simulink model "final_model"  (Simulink 10.0)
settings: Solver=VariableStepAuto  StartTime=0.0  StopTime=0.1  RelTol=1e-3
values from neighbouring files (symbols this model uses):
  Cth1 = 2.995e-4    (= 0.0002995)    [Initialization_naireeta.m]
  Cth2 = 0.0044    [Initialization_naireeta.m]
  Cth3 = 0.00376    [Initialization_naireeta.m]
  Irate = 10    [Initialization_naireeta.m]
  J = 1440    [Initialization_naireeta.m]
  Llrp = 0.00824    [Initialization_naireeta.m]
  Lls = 0.00103    [Initialization_naireeta.m]
  LM = 0.00639    [Initialization_naireeta.m]
  P = 4    [Initialization_naireeta.m]
  rrp = 2.25    [Initialization_naireeta.m]
  rs = 0.4    [Initialization_naireeta.m]
  Rth1 = 0.0850    (= 0.085)    [Initialization_naireeta.m]
  Rth2 = 0.353    [Initialization_naireeta.m]
  Rth3 = 0.7321    [Initialization_naireeta.m]
  Ts = 1e-6    (= 1e-06)    [Initialization_naireeta.m]
libraries: powerlib x135, powerlib_meascontrol x3, simulink x1
(part 2 of 2)

== system final_model/Thermal /Subsystem8 ==
  Ploss : Inport
  Ta : Inport  Port=2
  Controlled Current Source : powerlib/Electrical Sources/Controlled Current Source  Initialize=on  Source_Type=AC  Amplitude=0  Phase=0  Frequency=0  Measurements=None
      settings: SourceProductName=Simscape Electrical
  Controlled Voltage Source : powerlib/Electrical Sources/Controlled Voltage Source  Initialize=on  Source_Type=AC  Amplitude=0  Phase=0  Frequency=0  Measurements=None
      settings: SourceProductName=Simscape Electrical
  Series RLC Branch : powerlib/Elements/Series RLC Branch  LConnTagsString=__new0  RConnTagsString=__new0  BranchType=R  Resistance=Rth1  Inductance=1e-3  SetiL0=off  InitialCurrent=0  Capacitance=1e-6  Setx0=off  InitialVoltage=0  Measurements=None
      settings: SourceProductName=Simscape Electrical
  Series RLC Branch1 : powerlib/Elements/Series RLC Branch  LConnTagsString=__new0  RConnTagsString=__new0  BranchType=C  Resistance=1  Inductance=1e-3  SetiL0=off  InitialCurrent=0  Capacitance=Cth1  Setx0=off  InitialVoltage=0  Measurements=None
      settings: SourceProductName=Simscape Electrical
  Series RLC Branch2 : powerlib/Elements/Series RLC Branch  LConnTagsString=__new0  RConnTagsString=__new0  BranchType=R  Resistance=Rth2  Inductance=1e-3  SetiL0=off  InitialCurrent=0  Capacitance=1e-6  Setx0=off  InitialVoltage=0  Measurements=None
      settings: SourceProductName=Simscape Electrical
  Series RLC Branch3 : powerlib/Elements/Series RLC Branch  LConnTagsString=__new0  RConnTagsString=__new0  BranchType=C  Resistance=1  Inductance=1e-3  SetiL0=off  InitialCurrent=0  Capacitance=Cth2  Setx0=off  InitialVoltage=0  Measurements=None
      settings: SourceProductName=Simscape Electrical
  Series RLC Branch4 : powerlib/Elements/Series RLC Branch  LConnTagsString=__new0  RConnTagsString=__new0  BranchType=R  Resistance=Rth3  Inductance=1e-3  SetiL0=off  InitialCurrent=0  Capacitance=1e-6  Setx0=off  InitialVoltage=0  Measurements=None
      settings: SourceProductName=Simscape Electrical
  Series RLC Branch5 : powerlib/Elements/Series RLC Branch  LConnTagsString=__new0  RConnTagsString=__new0  BranchType=C  Resistance=1  Inductance=1e-3  SetiL0=off  InitialCurrent=0  Capacitance=Cth3  Setx0=off  InitialVoltage=0  Measurements=None
      settings: SourceProductName=Simscape Electrical
  Voltage Measurement : powerlib/Measurements/Voltage Measurement  PhasorSimulation=off  OutputType=Complex  PSBequivalent=0
      settings: SourceProductName=Simscape Electrical
  "TJ1 " : Outport
  wires:
  Ploss/1 -> Controlled Current Source/1
  Ta/1 -> Controlled Voltage Source/1
  Voltage Measurement/1 -> "TJ1 "/1
  connections:
  Series RLC Branch/LConn1 -- Series RLC Branch1/LConn1 -- Controlled Current Source/RConn1
  Series RLC Branch/RConn1 -- Voltage Measurement/LConn1 -- Series RLC Branch2/LConn1 -- Series RLC Branch3/LConn1 -- Series RLC Branch1/RConn1
  Controlled Voltage Source/LConn1 -- Voltage Measurement/LConn2 -- Controlled Current Source/LConn1
  Series RLC Branch4/LConn1 -- Series RLC Branch5/LConn1 -- Series RLC Branch2/RConn1 -- Series RLC Branch3/RConn1
  Series RLC Branch4/RConn1 -- Controlled Voltage Source/RConn1 -- Series RLC Branch5/RConn1

== system final_model/Thermal /Subsystem9 ==
  Ploss : Inport
  Ta : Inport  Port=2
  Controlled Current Source : powerlib/Electrical Sources/Controlled Current Source  Initialize=on  Source_Type=AC  Amplitude=0  Phase=0  Frequency=0  Measurements=None
      settings: SourceProductName=Simscape Electrical
  Controlled Voltage Source : powerlib/Electrical Sources/Controlled Voltage Source  Initialize=on  Source_Type=AC  Amplitude=0  Phase=0  Frequency=0  Measurements=None
      settings: SourceProductName=Simscape Electrical
  Series RLC Branch : powerlib/Elements/Series RLC Branch  LConnTagsString=__new0  RConnTagsString=__new0  BranchType=R  Resistance=Rth1  Inductance=1e-3  SetiL0=off  InitialCurrent=0  Capacitance=1e-6  Setx0=off  InitialVoltage=0  Measurements=None
      settings: SourceProductName=Simscape Electrical
  Series RLC Branch1 : powerlib/Elements/Series RLC Branch  LConnTagsString=__new0  RConnTagsString=__new0  BranchType=C  Resistance=1  Inductance=1e-3  SetiL0=off  InitialCurrent=0  Capacitance=Cth1  Setx0=off  InitialVoltage=0  Measurements=None
      settings: SourceProductName=Simscape Electrical
  Series RLC Branch2 : powerlib/Elements/Series RLC Branch  LConnTagsString=__new0  RConnTagsString=__new0  BranchType=R  Resistance=Rth2  Inductance=1e-3  SetiL0=off  InitialCurrent=0  Capacitance=1e-6  Setx0=off  InitialVoltage=0  Measurements=None
      settings: SourceProductName=Simscape Electrical
  Series RLC Branch3 : powerlib/Elements/Series RLC Branch  LConnTagsString=__new0  RConnTagsString=__new0  BranchType=C  Resistance=1  Inductance=1e-3  SetiL0=off  InitialCurrent=0  Capacitance=Cth2  Setx0=off  InitialVoltage=0  Measurements=None
      settings: SourceProductName=Simscape Electrical
  Series RLC Branch4 : powerlib/Elements/Series RLC Branch  LConnTagsString=__new0  RConnTagsString=__new0  BranchType=R  Resistance=Rth3  Inductance=1e-3  SetiL0=off  InitialCurrent=0  Capacitance=1e-6  Setx0=off  InitialVoltage=0  Measurements=None
      settings: SourceProductName=Simscape Electrical
  Series RLC Branch5 : powerlib/Elements/Series RLC Branch  LConnTagsString=__new0  RConnTagsString=__new0  BranchType=C  Resistance=1  Inductance=1e-3  SetiL0=off  InitialCurrent=0  Capacitance=Cth3  Setx0=off  InitialVoltage=0  Measurements=None
      settings: SourceProductName=Simscape Electrical
  Voltage Measurement : powerlib/Measurements/Voltage Measurement  PhasorSimulation=off  OutputType=Complex  PSBequivalent=0
      settings: SourceProductName=Simscape Electrical
  "TJ1 " : Outport
  wires:
  Ploss/1 -> Controlled Current Source/1
  Ta/1 -> Controlled Voltage Source/1
  Voltage Measurement/1 -> "TJ1 "/1
  connections:
  Series RLC Branch/LConn1 -- Series RLC Branch1/LConn1 -- Controlled Current Source/RConn1
  Series RLC Branch/RConn1 -- Voltage Measurement/LConn1 -- Series RLC Branch2/LConn1 -- Series RLC Branch3/LConn1 -- Series RLC Branch1/RConn1
  Controlled Voltage Source/LConn1 -- Voltage Measurement/LConn2 -- Controlled Current Source/LConn1
  Series RLC Branch4/LConn1 -- Series RLC Branch5/LConn1 -- Series RLC Branch2/RConn1 -- Series RLC Branch3/RConn1
  Series RLC Branch4/RConn1 -- Controlled Voltage Source/RConn1 -- Series RLC Branch5/RConn1

== system final_model/IM /Dynamic model of IM/Electromagnetic Torque ==
  Add : Sum  Inputs=+-
  Gain : Gain  Gain=(3/2)*(P/2)
  Product : Product  RndMeth=Zero
  Product1 : Product  RndMeth=Zero
  tag scope: Te=global
  wires:
  Add/1 -> Gain/1
  [lamda_ds] -> Product/1
  [iqs] -> Product/2
  [lamda_qs] -> Product1/1
  [ids] -> Product1/2
  Product/1 -> Add/1
  Product1/1 -> Add/2
  Gain/1 -> [Te]

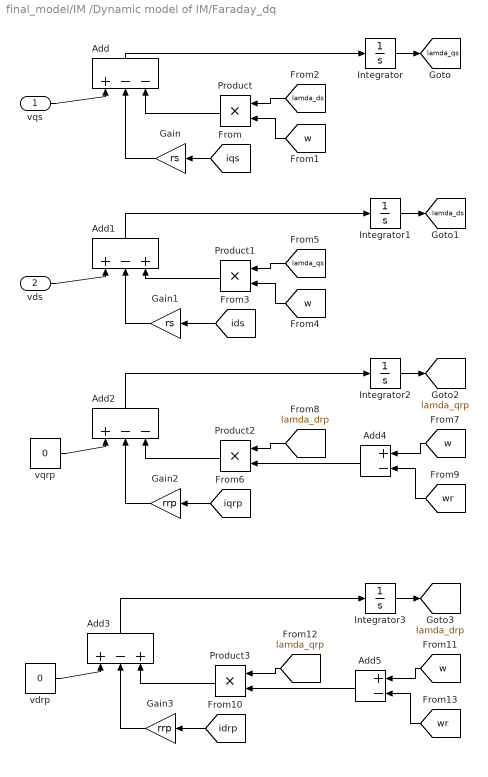
== system final_model/IM /Dynamic model of IM/Faraday_dq ==
  vqs : Inport
  vds : Inport  Port=2
  Add : Sum  Inputs=+--
  Add1 : Sum  Inputs=+-+
  Add2 : Sum  Inputs=+--
  Add3 : Sum  Inputs=+-+
  Add4 : Sum  Inputs=+-
  Add5 : Sum  Inputs=+-
  Gain : Gain  Gain=rs
  Gain1 : Gain  Gain=rs
  Gain2 : Gain  Gain=rrp
  Gain3 : Gain  Gain=rrp
  Integrator{,1..3} (4 alike) : Integrator
  Product{,1..3} (4 alike) : Product  RndMeth=Zero
  vdrp : Constant  Value=0
  vqrp : Constant  Value=0
  tag scope: lamda_drp=global, lamda_ds=global, lamda_qrp=global, lamda_qs=global
  wires:
  vqs/1 -> Add/1
  vds/1 -> Add1/1
  vqrp/1 -> Add2/1
  Gain/1 -> Add/2
  [iqs] -> Gain/1
  [w] -> Product/2
  [lamda_ds] -> Product/1
  Add/1 -> Integrator/1
  Product/1 -> Add/3
  Integrator/1 -> [lamda_qs]
  Gain1/1 -> Add1/2
  [ids] -> Gain1/1
  Integrator1/1 -> [lamda_ds]
  Add1/1 -> Integrator1/1
  [w] -> Product1/2
  [lamda_qs] -> Product1/1
  Product1/1 -> Add1/3
  Gain2/1 -> Add2/2
  [iqrp] -> Gain2/1
  [lamda_drp] -> Product2/1
  Product2/1 -> Add2/3
  [w] -> Add4/1
  [wr] -> Add4/2
  Add4/1 -> Product2/2
  Integrator2/1 -> [lamda_qrp]
  Add2/1 -> Integrator2/1
  vdrp/1 -> Add3/1
  Gain3/1 -> Add3/2
  [idrp] -> Gain3/1
  [lamda_qrp] -> Product3/1
  Product3/1 -> Add3/3
  [w] -> Add5/1
  [wr] -> Add5/2
  Add5/1 -> Product3/2
  Integrator3/1 -> [lamda_drp]
  Add3/1 -> Integrator3/1

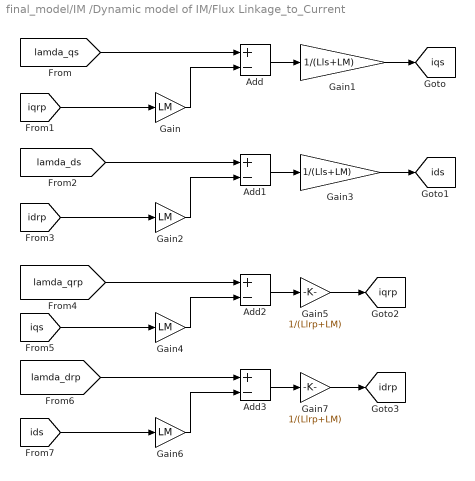
== system final_model/IM /Dynamic model of IM/Flux Linkage_to_Current ==
  Add{,1..3} (4 alike) : Sum  Inputs=+-
  Gain{,2,4,6} (4 alike) : Gain  Gain=LM
  Gain1 : Gain  Gain=1/(Lls+LM)
  Gain3 : Gain  Gain=1/(Lls+LM)
  Gain5 : Gain  Gain=1/(Llrp+LM)
  Gain7 : Gain  Gain=1/(Llrp+LM)
  tag scope: idrp=global, ids=global, iqrp=global, iqs=global
  wires:
  [lamda_qs] -> Add/1
  Gain/1 -> Add/2
  Add/1 -> Gain1/1
  Gain1/1 -> [iqs]
  [iqrp] -> Gain/1
  [lamda_ds] -> Add1/1
  Gain2/1 -> Add1/2
  Add1/1 -> Gain3/1
  Gain3/1 -> [ids]
  [idrp] -> Gain2/1
  [lamda_qrp] -> Add2/1
  Gain4/1 -> Add2/2
  Add2/1 -> Gain5/1
  Gain5/1 -> [iqrp]
  [iqs] -> Gain4/1
  [lamda_drp] -> Add3/1
  Gain6/1 -> Add3/2
  Add3/1 -> Gain7/1
  Gain7/1 -> [idrp]
  [ids] -> Gain6/1

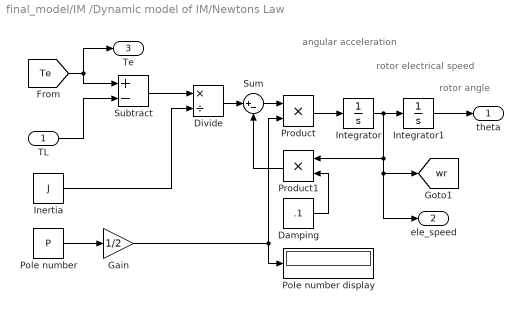
== system final_model/IM /Dynamic model of IM/Newtons Law ==
  note: rotor
      | angle
  note: rotor
      | electrical
      | speed
  note: angular
      | acceleration
  TL : Inport
  Damping : Constant  Value=.1
  Divide : Product  Inputs=*/
  Gain : Gain  Gain=1/2
  Inertia : Constant  Value=J
  Integrator : Integrator
  Integrator1 : Integrator
  Pole number : Constant  Value=P
  Pole number display : Display
  Product : Product  RndMeth=Zero
  Product1 : Product  RndMeth=Zero
  Subtract : Sum  Inputs=+-
  Sum : Sum  Inputs=|+-
  theta : Outport
  ele_speed : Outport  Port=2
  Te : Outport  Port=3
  tag scope: wr=global
  wires:
  [Te] -> Subtract/1, Te/1
  TL/1 -> Subtract/2
  Subtract/1 -> Divide/1
  Inertia/1 -> Divide/2
  Pole number/1 -> Gain/1
  Gain/1 -> Product/2, Pole number display/1
  Product/1 -> Integrator/1
  Integrator/1 -> Integrator1/1, Product1/1, ele_speed/1, [wr]
  Integrator1/1 -> theta/1
  Damping/1 -> Product1/2
  Divide/1 -> Sum/1
  Sum/1 -> Product/1
  Product1/1 -> Sum/2

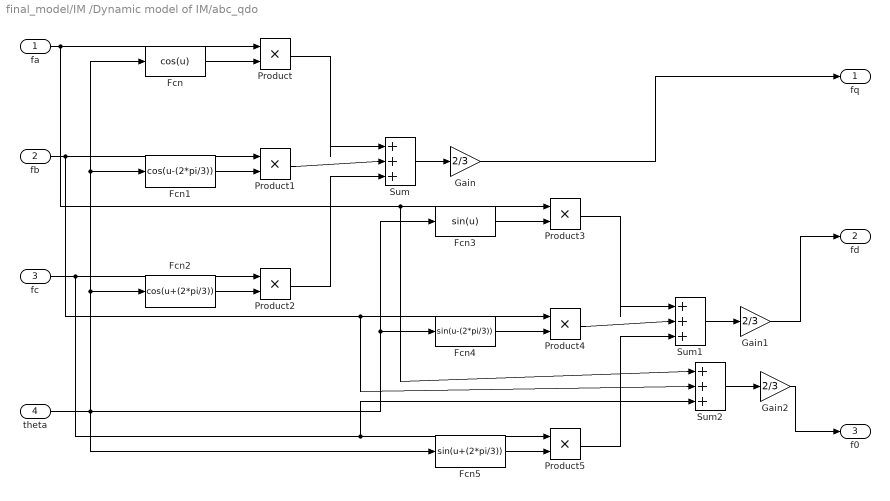
== system final_model/IM /Dynamic model of IM/abc_qdo ==
  fa : Inport
  fb : Inport  Port=2
  fc : Inport  Port=3
  theta : Inport  Port=4
  Fcn : Fcn  Expr=cos(u)
  Fcn1 : Fcn  Expr=cos(u-(2*pi/3))
  Fcn2 : Fcn  Expr=cos(u+(2*pi/3))
  Fcn3 : Fcn  Expr=sin(u)
  Fcn4 : Fcn  Expr=sin(u-(2*pi/3))
  Fcn5 : Fcn  Expr=sin(u+(2*pi/3))
  Gain : Gain  Gain=2/3
  Gain1 : Gain  Gain=2/3
  Gain2 : Gain  Gain=2/3
  Product{,1..5} (6 alike) : Product  RndMeth=Zero
  Sum : Sum  Inputs=|+++
  Sum1 : Sum  Inputs=|+++
  Sum2 : Sum  Inputs=|+++
  fq : Outport
  fd : Outport  Port=2
  f0 : Outport  Port=3
  wires:
  Fcn/1 -> Product/2
  fa/1 -> Product/1, Product3/1, Sum2/1
  fb/1 -> Product1/1, Product4/1, Sum2/2
  Fcn1/1 -> Product1/2
  fc/1 -> Product2/1, Product5/1, Sum2/3
  Fcn2/1 -> Product2/2
  Product/1 -> Sum/1
  Product1/1 -> Sum/2
  Product2/1 -> Sum/3
  Sum/1 -> Gain/1
  theta/1 -> Fcn2/1, Fcn1/1, Fcn/1, Fcn5/1, Fcn3/1, Fcn4/1
  Gain/1 -> fq/1
  Fcn3/1 -> Product3/2
  Fcn4/1 -> Product4/2
  Fcn5/1 -> Product5/2
  Product3/1 -> Sum1/1
  Product4/1 -> Sum1/2
  Product5/1 -> Sum1/3
  Sum1/1 -> Gain1/1
  Gain1/1 -> fd/1
  Sum2/1 -> Gain2/1
  Gain2/1 -> f0/1

== matlab function SBC ==
  data: i_ref input double; fsw output double; Vab0 input double; Iab0 input double; Irate input double; Vdc input double; R input double; L input double; Tsw input double; P_loss output double size=[1 12]; Th_en input double; Sequence output double; State_p input double; TJ input double; T_out input double
function [fsw,P_loss,Sequence]  = fcn(i_ref,Vab0,Iab0,Irate,Vdc,R,L,Tsw,Th_en,State_p,TJ,T_out)
M_ab=[1 0 1;
      -0.5 sqrt(3)/2 1;
      -0.5 -sqrt(3)/2 1];
SwitchSequence = [-1 -1 -1; 0 0 0; 1 1 1; 1 0 0; 0 -1 -1; 0 0 -1; 1 1 0; 0 1 0; -1 0 -1; -1 0 0;...
    0 1 1; 0 0 1; -1 -1 0; 0 -1 0; 1 0 1; 1 -1 -1; 1 0 -1; 1 1 -1; 0 1 -1; -1 1 -1; -1 1 0;...
    -1 1 1; -1 0 1; -1 -1 1; 0 -1 1; 1 -1 1; 1 -1 0];
SwitchCommand = [0 0 1 1 0 0 1 1 0 0 1 1; 0 1 1 0 0 1 1 0 0 1 1 0; 1 1 0 0 1 1 0 0 1 1 0 0;...
    1 1 0 0 0 1 1 0 0 1 1 0; 0 1 1 0 0 0 1 1 0 0 1 1;0 1 1 0 0 1 1 0 0 0 1 1; 1 1 0 0 1 1 0 0 0 1 1 0;...
    0 1 1 0 1 1 0 0 0 1 1 0; 0 0 1 1 0 1 1 0 0 0 1 1; 0 0 1 1 0 1 1 0 0 1 1 0; 0 1 1 0 1 1 0 0 1 1 0 0;...
    0 1 1 0 0 1 1 0 1 1 0 0;
    0 0 1 1 0 0 1 1 0 1 1 0;0 1 1 0 0 0 1 1 0 1 1 0; 1 1 0 0 0 1 1 0 1 1 0 0;...
    1 1 0 0 0 0 1 1 0 0 1 1; 1 1 0 0 0 1 1 0 0 0 1 1; 1 1 0 0 1 1 0 0 0 0 1 1; 0 1 1 0 1 1 0 0 0 0 1 1;...
    0 0 1 1 1 1 0 0 0 0 1 1; 0 0 1 1 1 1 0 0 0 1 1 0;
    0 0 1 1 1 1 0 0 1 1 0 0; 0 0 1 1 0 1 1 0 1 1 0 0; 0 0 1 1 0 0 1 1 1 1 0 0;...
    0 1 1 0 0 0 1 1 1 1 0 0; 1 1 0 0 0 0 1 1 1 1 0 0; 1 1 0 0 0 0 1 1 0 1 1 0];
vSequence=Vdc/3*[0 0 0 ;0 0 0; 0 0 0;  1 0 0; 1 0 0; 1/2 sqrt(3)/2 0; 1/2 sqrt(3)/2 0;...
    -1/2 sqrt(3)/2 0; -1/2 sqrt(3)/2 0; -1 0 0; -1 0 0; -1/2 -sqrt(3)/2 0; -1/2 -sqrt(3)/2 0; 1/2 -sqrt(3)/2 0;...
    1/2 -sqrt(3)/2 0; 2 0 0; 3/2 sqrt(3)/2 0; 1 sqrt(3) 0; 0 sqrt(3) 0; -1 sqrt(3) 0; -3/2 sqrt(3)/2 0; -2 0 0;...
    -3/2 -sqrt(3)/2 0; -1 -sqrt(3) 0; 0 -sqrt(3) 0; 1 -sqrt(3) 0; 3/2 -sqrt(3)/2 0];
Jp=inf;
Sequence=1;
m=0.4;
i_sbc=zeros(3,1);
i_tmp = zeros(3,1);
E_con_MOS=zeros(1,12);
E_con_D=zeros(1,12);
E_swt_MOS=zeros(1,12);
E_swt_D=zeros(1,12);
E_swt_MOS=zeros(1,12);
E_swt_D=zeros(1,12);
P_loss=zeros(1,12);
E_loss1 = 0;
E_loss2 = 0;
E_loss3 = 0;
Jx=zeros(27,1);
w_e=0.5;%0.94; %Electrical cost weight
w_th=1-w_e; %Thermal cost weight
E_rate=60e-3; %Rated Switching losses 3*(2.8+2.19+1)

for k=1:27
    itmp_alpha=(L/(L+R*Tsw)*Iab0(1))+(Tsw/(L+R*Tsw)*vSequence(k,1));
    itmp_beta=(L/(L+R*Tsw)*Iab0(2))+(Tsw/(L+R*Tsw)*vSequence(k,2));
    Je=((i_ref(1)-itmp_alpha)/Irate)^2+((i_ref(2)-itmp_beta)/Irate)^2; % Electrical system cost functine
    Jx(k)=Je;
    
    if Th_en == 1
        E_con_MOS=zeros(1,12);
        E_con_D=zeros(1,12);
        E_swt_MOS=zeros(1,12);
        E_swt_D=zeros(1,12);
        
        % abc current
        i_tmp=M_ab*[itmp_alpha;itmp_beta;Iab0(3)];
        
        %% Calculation of conduction losses
        %Phase A
        if SwitchSequence(k,1)==1
            if i_tmp(1)>=0
                E_con_D(1)=m*abs(i_tmp(1))*2*Tsw;
                E_con_D(2)=m*abs(i_tmp(1))*2*Tsw;
            else
                E_con_MOS(3)=(1-m)*abs(i_tmp(1))*2*Tsw;
                E_con_MOS(4)=(1-m)*abs(i_tmp(1))*2*Tsw;
            end
        else
            if i_tmp(1)<=0
                E_con_D(3)=m*abs(i_tmp(1))*2*Tsw;
                E_con_D(4)=m*abs(i_tmp(1))*2*Tsw;
            else
                E_con_MOS(1)=(1-m)*abs(i_tmp(1))*2*Tsw;
                E_con_MOS(2)=(1-m)*abs(i_tmp(1))*2*Tsw;
            end
        end
        
        %Phase B
        if SwitchSequence(k,2)==1
            if i_tmp(2)>=0
                E_con_D(5)=m*abs(i_tmp(2))*2*Tsw;
                E_con_D(6)=m*abs(i_tmp(2))*2*Tsw;
            else
                E_con_MOS(7)=(1-m)*abs(i_tmp(2))*2*Tsw;
                E_con_MOS(8)=(1-m)*abs(i_tmp(2))*2*Tsw;
            end

            if i_tmp(2)<=0
                E_con_D(7)=m*abs(i_tmp(2))*2*Tsw;
                E_con_D(8)=m*abs(i_tmp(2))*2*Tsw;
            else
                E_con_MOS(5)=(1-m)*abs(i_tmp(2))*2*Tsw;
                E_con_MOS(6)=(1-m)*abs(i_tmp(2))*2*Tsw;
            end
        end
        
        %Phase C
        if SwitchSequence(k,3)==1
            if i_tmp(3)>=0
                E_con_D(9)=m*abs(i_tmp(3))*2*Tsw;
                E_con_D(10)=m*abs(i_tmp(3))*2*Tsw;
            else
                E_con_MOS(11)=(1-m)*abs(i_tmp(3))*2*Tsw;
                E_con_MOS(12)=(1-m)*abs(i_tmp(3))*2*Tsw;
            end
        else
            if i_tmp(2)<=0
                E_con_D(11)=m*abs(i_tmp(3))*2*Tsw;
                E_con_D(12)=m*abs(i_tmp(3))*2*Tsw;
            else
                E_con_MOS(9)=(1-m)*abs(i_tmp(3))*2*Tsw;
                E_con_MOS(10)=(1-m)*abs(i_tmp(3))*2*Tsw;
            end
        end
        
        %% Switching Losses
        % Leg A
        if SwitchSequence(State_p, 1) == SwitchSequence(k, 1)
            E_swt_MOS(1) = 0;
            E_swt_MOS(2) = 0;
            E_swt_MOS(3) = 0;
            E_swt_MOS(4) = 0;
            E_swt_D(1) = 0;
            E_swt_D(2) = 0;
            E_swt_D(3) = 0;
            E_swt_D(4) = 0;
            E_loss1 = 0;
        else
            E_on_2=(0.0345*abs(i_tmp(1))+0.05)*1e-3*abs(Vdc)/600;
            E_off_2=(0.0566*abs(i_tmp(1))+0.24)*1e-3*abs(Vdc)/600;
            E_rr_2=(0.04*abs(i_tmp(1))+0.51)*1e-3*abs(Vdc)/600;
            if SwitchSequence(k, 1) == 1
                if i_tmp(1) >= 0
                    E_swt_MOS(3) = E_off_2;
                    E_swt_MOS(4) = E_off_2;
                else
                    E_swt_MOS(1) = E_on_2;
                    E_swt_MOS(2) = E_on_2;
                    E_swt_D(3) = E_rr_2;
                    E_swt_D(4) = E_rr_2;
                end
            else
                if i_tmp(1) >= 0
                    E_swt_MOS(3) = E_on_2;
                    E_swt_MOS(4) = E_on_2;
                    E_swt_D(1) = E_rr_2;
                    E_swt_D(2) = E_rr_2;
                else
                    E_swt_MOS(1) = E_off_2;
                    E_swt_MOS(2) = E_off_2;
                end
            end
            
            E_loss1 = E_on_2 + E_off_2 + E_rr_2;
        end
        
        % Leg B
        if SwitchSequence(State_p, 2) == SwitchSequence(k, 2)
            E_swt_MOS(5) = 0;
            E_swt_MOS(6) = 0;
            E_swt_MOS(7) = 0;
            E_swt_MOS(8) = 0;
            E_swt_D(5) = 0;
            E_swt_D(6) = 0;
            E_swt_D(7) = 0;
            E_swt_D(8) = 0;
            E_loss2 = 0;
        else
            E_on_2=(0.0345*abs(i_tmp(1))+0.05)*1e-3*abs(Vdc)/600;
            E_off_2=(0.0566*abs(i_tmp(1))+0.24)*1e-3*abs(Vdc)/600;
            E_rr_2=(0.04*abs(i_tmp(1))+0.51)*1e-3*abs(Vdc)/600;
            
            if SwitchSequence(k, 2) == 1
                if i_tmp(2) >= 0
                    E_swt_MOS(7) = E_off_2;
                    E_swt_MOS(8) = E_off_2;
                else
                    E_swt_MOS(5)=E_on_2;
                    E_swt_MOS(6)=E_on_2;
                    E_swt_D(7)=E_rr_2;
                    E_swt_D(8)=E_rr_2;
                end
            else
                if i_tmp(2) >= 0
                    E_swt_MOS(7)=E_on_2;
                    E_swt_MOS(8)=E_on_2;
                    E_swt_D(5)=E_rr_2;
                    E_swt_D(6)=E_rr_2;
                else
                    E_swt_MOS(5)=E_off_2;
                    E_swt_MOS(6)=E_off_2;
                end
            end
            
            E_loss2 = E_on_2 + E_off_2 + E_rr_2;
        end
        
        % Leg C
        if SwitchSequence(State_p,3)==SwitchSequence(k,3)
            E_swt_MOS(9)=0;
            E_swt_MOS(10)=0;
            E_swt_MOS(11)=0;
            E_swt_MOS(12)=0;
            E_swt_D(9)=0;
            E_swt_D(10)=0;
            E_swt_D(11)=0;
            E_swt_D(12)=0;
            E_loss3=0;
        else
              E_on_3=(0.0345*abs(i_tmp(1))+0.05)*1e-3*abs(Vdc)/600;
            E_off_3=(0.0566*abs(i_tmp(1))+0.24)*1e-3*abs(Vdc)/600;
            E_rr_3=(0.04*abs(i_tmp(1))+0.51)*1e-3*abs(Vdc)/600;
            if SwitchSequence(k,3)==1
                if i_tmp(3)>=0
                    E_swt_MOS(11)=E_off_3;
                    E_swt_MOS(12)=E_off_3;
                else
                    E_swt_MOS(9)=E_on_3;
                    E_swt_MOS(10)=E_on_3;
                    E_swt_D(11)=E_rr_3;
                    E_swt_D(12)=E_rr_3;
                end
            else
                if i_tmp(3)>=0
                    E_swt_MOS(11)=E_on_3;
                    E_swt_MOS(12)=E_on_3;
                    E_swt_D(9)=E_rr_3;
                    E_swt_D(10)=E_rr_3;
                else
                    E_swt_MOS(9)=E_off_3;
                    E_swt_MOS(10)=E_off_3;
                end
            end
            
            E_loss3=E_on_3+E_off_3+E_rr_3;
        end
        
        E_loss = (E_loss1 + E_loss2 + E_loss3);
        J_th = (E_loss/E_rate)^2;
        J=w_e*Je+w_th*abs(0.008-J_th);
        if J < Jp
            Jp = J;
            Sequence = k;
            Loss = E_loss;
            i_sbc = i_tmp;
            P_loss = [E_con_MOS + E_swt_MOS + E_con_D + E_swt_D]/Tsw;
        end
    else
        if Je < Jp
            Jp = Je;
            Sequence=k;
            i_sbc = [itmp_alpha; itmp_beta; 0];
        end
        P_loss = zeros(1, 12);
    end
    
    fsw=SwitchCommand(Sequence,:)';
end
